simulink model "ViscoelasticBodies"  (R2025b)
settings: Solver=VariableStepAuto  StartTime=0.0  StopTime=10.0  RelTol=1e-3
undefined symbols (not defined in the file): sigbuilder_block
libraries: simulink x2
settings Model: Creator=ARDA  LastModifiedBy=carla
settings DebuggingCC: UnconnectedInputMsg=warning  UnconnectedOutputMsg=warning  UnconnectedLineMsg=warning
settings ModelReferenceCC: EnableRefExpFcnMdlSchedulingChecks=on
settings RTWCC: GPUComputeCapability=3.5  DLArmComputeVersion=19.05

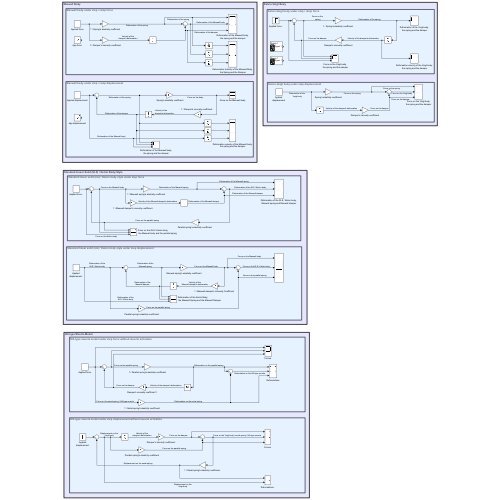
[thumbnail: Simulink's stored preview of the top-level diagram]
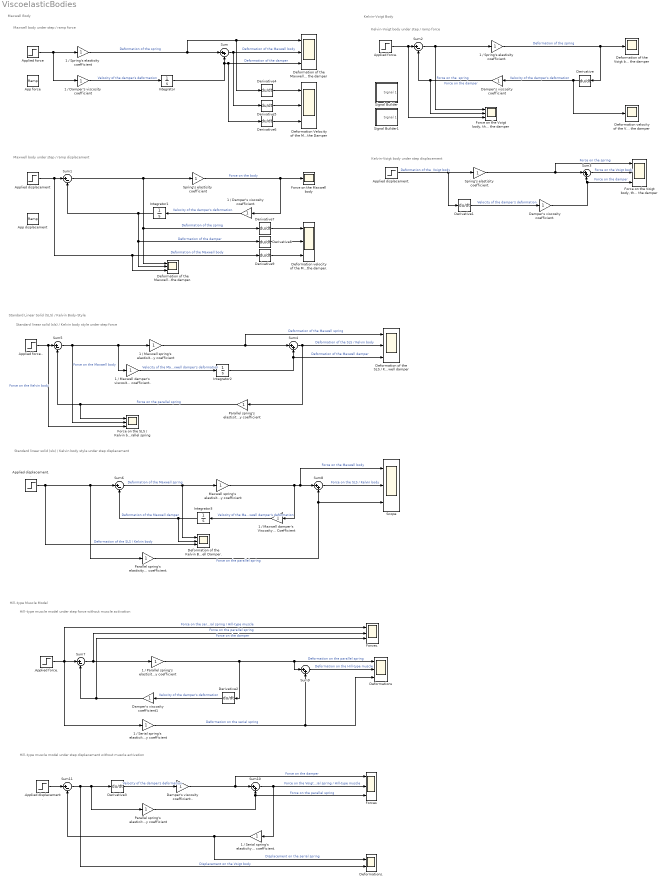
== system ViscoelasticBodies ==
  note: Hill-type Muscle Model
  note: Hill-type muscle model under step displacement without muscle activation
  note: Hill-type muscle model under step force without muscle activation
  note: Standard Linear Solid (SLS) / Kelvin Body-Style
  note: Standard linear solid (sls) / Kelvin body style under step displacement
  note: Standard linear solid (sls) / Kelvin body style under step force
  note: Kelvin-Voigt Body
  note: Kelvin-Voigt body under step displacement
  note: Kelvin-Voigt body under step / ramp force
  note: Maxwell Body
  note: Maxwell body under step / ramp displacement
  note: Maxwell body under step / ramp force
  .Applied displacement. : Step  SampleTime=0
  .Applied force. : Step  SampleTime=0
  1 / Damper's viscosity coefficient : Gain
  1 / Damper's viscosity coefficient. : Gain
  1 / Maxwell damper's Viscosity Coefficient : Gain
  1 / Maxwell damper's viscosity coefficient.. : Gain
  1 / Maxwell spring's elastisity coefficient : Gain
  1 / Parallel spring's elastisity coefficient : Gain
  1 / Serial spring's elasticity coefficient : Gain
  1 / Serial spring's elasticity coefficient. : Gain
  1 / Spring's elastisity coefficient : Gain
  1 / Spring's elastisity coefficient. : Gain
  App displacement : simulink/Sources/Ramp  slope=1  start=0  InitialOutput=0
  App force : simulink/Sources/Ramp  slope=1  start=0  InitialOutput=0
  Applied displacement. : Step  SampleTime=0
  Applied displacement.. : Step  SampleTime=0
  Applied displacement : Step  SampleTime=0
  Applied force : Step  SampleTime=0
  Applied force. : Step  SampleTime=0
  Applied force.. : Step  SampleTime=0
  Damper's viscosity coefficient : Gain
  Damper's viscosity coefficient. : Gain
  Damper's viscosity coefficient.. : Gain
  Damper's viscosity coefficient1 : Gain
  "Deformation Velocity of the Maxwell Body, the Spring and the Damper" : Scope  NumInputPorts=3
      settings: ActiveDisplayYMinimum=-1.7592186044415996E+13  ActiveDisplayYMaximum=1.58329674399744E+14
  "Deformation of the Kelvin Body, the Maxwell Spring and the Maxwell Damper." : Scope  NumInputPorts=3
      settings: ActiveDisplayYMinimum=-0.12499999999999997  ActiveDisplayYMaximum=1.125  DataLoggingVariableName=ScopeData8
  "Deformation of the Maxwell body, the spring and the damper" : Scope  NumInputPorts=3
      settings: ActiveDisplayYMinimum=-1.25  ActiveDisplayYMaximum=11.250000000000002
  "Deformation of the Maxwell body, the spring and the damper." : Scope  NumInputPorts=3
      settings: ActiveDisplayYMinimum=-0.12499999999999997  ActiveDisplayYMaximum=1.125  DataLoggingVariableName=ScopeData3
  "Deformation of the SLS / Kelvin body, Maxwell spring and Maxwell damper" : Scope  NumInputPorts=3
      settings: ActiveDisplayYMinimum=-0.12430568770609152  ActiveDisplayYMaximum=1.1187511893548239  DataLoggingVariableName=ScopeData6
  "Deformation of the Voigt body, the spring and the damper" : Scope
      settings: ActiveDisplayYMinimum=-0.12496582142586175  ActiveDisplayYMaximum=1.1246923928327561  DataLoggingVariableName=ScopeData2
  "Deformation velocity of the Maxwell body, the spring and the damper." : Scope  NumInputPorts=3
      settings: ActiveDisplayYMinimum=-1.7592186044417121E+13  ActiveDisplayYMaximum=1.5832967439974412E+14  DataLoggingVariableName=ScopeData2
  "Deformation velocity of the Voigt body, the spring and the damper" : Scope
      settings: ActiveDisplayYMinimum=-0.57803031764403257  ActiveDisplayYMaximum=0.67102285879629342
  Deformations : Scope  NumInputPorts=3
      settings: ActiveDisplayYMinimum=-0.24996582142586171  ActiveDisplayYMaximum=2.2496923928327561  DataLoggingVariableName=ScopeData2
  Deformations. : Scope  NumInputPorts=2
      settings: ActiveDisplayYMinimum=-0.12499999999999908  ActiveDisplayYMaximum=1.124999999999992
  Derivative{,1..9} (10 alike) : Derivative
  Force on the Maxwell body : Scope
      settings: ActiveDisplayYMinimum=-0.12499999999999997  ActiveDisplayYMaximum=1.125
  "Force on the SLS / Kelvin body, the Maxwell body and the parallel spring" : Scope  NumInputPorts=3
      settings: ActiveDisplayYMinimum=-0.125  ActiveDisplayYMaximum=1.125  DataLoggingVariableName=ScopeData7
  "Force on the Voigt body, the spring and the damper" : Scope  NumInputPorts=3
      settings: ActiveDisplayYMinimum=-0.66553  ActiveDisplayYMaximum=1.18506  DataLoggingVariableName=ScopeData4
  "Force on the Voigt body, the spring and the damper" : Scope  NumInputPorts=3
      settings: ActiveDisplayYMinimum=-1.7592186044416121E+13  ActiveDisplayYMaximum=1.5832967439974512E+14  DataLoggingVariableName=ScopeData5
  Forces : Scope  NumInputPorts=3
      settings: ActiveDisplayYMinimum=-0.12499999999999908  ActiveDisplayYMaximum=1.124999999999992  DataLoggingVariableName=ScopeData2
  Forces. : Scope  NumInputPorts=3
      settings: ActiveDisplayYMinimum=-0.12499999999999997  ActiveDisplayYMaximum=1.125  DataLoggingVariableName=ScopeData3
  Integrator{,1..3} (4 alike) : Integrator
  Maxwell spring's elastisity coefficient : Gain
  Parallel spring's elasticity coefficient : Gain
  Parallel spring's elastisity coefficient : Gain
  Parallel spring's elastisity coefficient. : Gain
  Scope : Scope  NumInputPorts=3
      settings: ActiveDisplayYMinimum=-0.24999999999999994  ActiveDisplayYMaximum=2.25  DataLoggingVariableName=ScopeData9
  Signal Builder : Subsystem  Tag=STV Subsys  LoadFcn=sigbuilder_block('load');  StartFcn=sigbuilder_block('start');  StopFcn=sigbuilder_block('stop');  ClipboardFcn=sigbuilder_block('clipboard');  mask(Sigbuilder block){tuvar=[0:10]}
      mask help: Simulink:masks:SigbuilderBlock_MD
      mask init:
      | if ~strcmp(get_param(bdroot(gcbh),'SimulationStatus'),'stopped') tuvar = sigbuilder_block('maskInit'); end
      settings: CopyFcn=sigbuilder_block('copy');  DeleteFcn=sigbuilder_block('delete');  ModelCloseFcn=sigbuilder_block('modelClose');  PreSaveFcn=sigbuilder_block('preSave');  PauseFcn=sigbuilder_block('pause');  ContinueFcn=sigbuilder_block('continue');  NameChangeFcn=sigbuilder_block('namechange');  OpenFcn=sigbuilder_block('open',[316.5 171.75 805.5 485.25 ]);  CloseFcn=sigbuilder_block('close');
      mask Display: plot(0, 0, 100, 100,[2, 2, 32, 32, 2], [68, 8, 8, 68, 68],[32, 2], [38, 38], [32, 19, 2],[53, 60, 44], [32, 17, 17, 2],[16, 16, 31, 31]);txt = getActiveGroup(gcbh);text(2, 100, txt,'verticalAlignment', 'top');
  Signal Builder1 : Subsystem  Tag=STV Subsys  LoadFcn=sigbuilder_block('load');  StartFcn=sigbuilder_block('start');  StopFcn=sigbuilder_block('stop');  ClipboardFcn=sigbuilder_block('clipboard');  mask(Sigbuilder block){tuvar=[0:10]}
      mask help: Simulink:masks:SigbuilderBlock_MD
      mask init:
      | if ~strcmp(get_param(bdroot(gcbh),'SimulationStatus'),'stopped') tuvar = sigbuilder_block('maskInit'); end
      settings: CopyFcn=sigbuilder_block('copy');  DeleteFcn=sigbuilder_block('delete');  ModelCloseFcn=sigbuilder_block('modelClose');  PreSaveFcn=sigbuilder_block('preSave');  PauseFcn=sigbuilder_block('pause');  ContinueFcn=sigbuilder_block('continue');  NameChangeFcn=sigbuilder_block('namechange');  OpenFcn=sigbuilder_block('open',[2397 1214.25 805.5 485.25 ]);  CloseFcn=sigbuilder_block('close');
      mask Display: plot(0, 0, 100, 100,[2, 2, 32, 32, 2], [68, 8, 8, 68, 68],[32, 2], [38, 38], [32, 19, 2],[53, 60, 44], [32, 17, 17, 2],[16, 16, 31, 31]);txt = getActiveGroup(gcbh);text(2, 100, txt,'verticalAlignment', 'top');
  Spring's elastisity coefficient : Gain
  Spring's elastisity coefficient. : Gain
  Sum{,3..4,8..10} (6 alike) : Sum  Inputs=|++
  Sum{1..2,5..7,11} (6 alike) : Sum  Inputs=|+-
  wires:
  Applied force/1 -> 1 / Damper's viscosity coefficient/1, 1 / Spring's elastisity coefficient/1
  1 / Damper's viscosity coefficient/1 -> Integrator/1  "Velocity of the damper's deformation"
  1 / Spring's elastisity coefficient/1 -> Derivative4/1, "Deformation of the Maxwell body, the spring and the damper"/1, Sum/1  "Deformation of the spring"
  Integrator/1 -> Derivative6/1, "Deformation of the Maxwell body, the spring and the damper"/3, Sum/2  "Deformation of the damper"
  Applied displacement/1 -> "Deformation of the Maxwell body, the spring and the damper."/3, Derivative9/1, Sum1/1  "Deformation of the Maxwell body"
  Sum1/1 -> Spring's elastisity coefficient/1, Derivative7/1, "Deformation of the Maxwell body, the spring and the damper."/1  "Deformation of the spring"
  Spring's elastisity coefficient/1 -> Force on the Maxwell body/1, 1 / Damper's viscosity coefficient./1  "Force on the body"
  1 / Damper's viscosity coefficient./1 -> Integrator1/1  "Velocity of the damper's deformation."
  Integrator1/1 -> Derivative8/1, "Deformation of the Maxwell body, the spring and the damper."/2, Sum1/2  "Deformation of the damper"
  Sum/1 -> Derivative5/1, "Deformation of the Maxwell body, the spring and the damper"/2  "Deformation of the Maxwell body"
  Applied force./1 -> "Force on the Voigt body, the spring and the damper"/3, Sum2/1
  Sum2/1 -> "Force on the Voigt body, the spring and the damper"/1, 1 / Spring's elastisity coefficient./1  "Force on the  spring"
  Damper's viscosity coefficient/1 -> Sum2/2, "Force on the Voigt body, the spring and the damper"/2  "Force on the damper"
  1 / Spring's elastisity coefficient./1 -> Derivative/1, "Deformation of the Voigt body, the spring and the damper"/1  "Deformation of the spring"
  Derivative/1 -> Damper's viscosity coefficient/1, "Deformation velocity of the Voigt body, the spring and the damper"/1  "Velocity of the damper's deformation"
  Applied displacement./1 -> Spring's elastisity coefficient./1, Derivative1/1  "Deformation of the  Voigt body"
  Derivative1/1 -> Damper's viscosity coefficient./1  "Velocity of the damper's deformation"
  Spring's elastisity coefficient./1 -> "Force on the Voigt body, the spring and the damper"/1, Sum3/1  "Force on the spring"
  Damper's viscosity coefficient./1 -> "Force on the Voigt body, the spring and the damper"/3, Sum3/2  "Force on the damper"
  Sum3/1 -> "Force on the Voigt body, the spring and the damper"/2  "Force on the Voigt body"
  Sum4/1 -> "Deformation of the SLS / Kelvin body, Maxwell spring and Maxwell damper"/2, Parallel spring's elastisity coefficient/1  "Deformation of the SLS / Kelvin body"
  Integrator2/1 -> "Deformation of the SLS / Kelvin body, Maxwell spring and Maxwell damper"/3, Sum4/2  "Deformation of the Maxwell damper"
  1 / Maxwell spring's elastisity coefficient/1 -> Sum4/1, "Deformation of the SLS / Kelvin body, Maxwell spring and Maxwell damper"/1  "Deformation of the Maxwell spring"
  1 / Maxwell damper's viscosity coefficient../1 -> Integrator2/1  "Velocity of the Maxwell damper's deformation"
  Sum5/1 -> "Force on the SLS / Kelvin body, the Maxwell body and the parallel spring"/2, 1 / Maxwell spring's elastisity coefficient/1, 1 / Maxwell damper's viscosity coefficient../1  "Force on the Maxwell body"
  Applied force../1 -> "Force on the SLS / Kelvin body, the Maxwell body and the parallel spring"/3, Sum5/1  "Force on the Kelvin body"
  Parallel spring's elastisity coefficient/1 -> "Force on the SLS / Kelvin body, the Maxwell body and the parallel spring"/1, Sum5/2  "Force on the parallel spring"
  Integrator3/1 -> "Deformation of the Kelvin Body, the Maxwell Spring and the Maxwell Damper."/2, Sum6/2  "Deformation of the Maxwell damper"
  1 / Maxwell damper's Viscosity Coefficient/1 -> Integrator3/1  "Velocity of the Maxwell damper's deformation"
  Maxwell spring's elastisity coefficient/1 -> Sum8/1, Scope/1, 1 / Maxwell damper's Viscosity Coefficient/1  "Force on the Maxwell body"
  Sum6/1 -> Maxwell spring's elastisity coefficient/1, "Deformation of the Kelvin Body, the Maxwell Spring and the Maxwell Damper."/1  "Deformation of the Maxwell spring"
  Applied displacement../1 -> Sum6/1, Parallel spring's elastisity coefficient./1, "Deformation of the Kelvin Body, the Maxwell Spring and the Maxwell Damper."/3  "Deformation of the SLS / Kelvin body"
  Parallel spring's elastisity coefficient./1 -> Scope/3, Sum8/2  "Force on the parallel spring"
  Sum8/1 -> Scope/2  "Force on the SLS / Kelvin body"
  Sum9/1 -> Deformations/2  "Deformation on the Hill-type muscle"
  Derivative2/1 -> Damper's viscosity coefficient1/1  "Velocity of the damper's deformation"
  1 / Parallel spring's elastisity coefficient/1 -> Sum9/1, Deformations/1, Derivative2/1  "Deformation on the parallel spring"
  1 / Serial spring's elasticity coefficient/1 -> Sum9/2, Deformations/3  "Deformation on the serial spring"
  Sum7/1 -> Forces./2, 1 / Parallel spring's elastisity coefficient/1  "Force on the parallel spring"
  Damper's viscosity coefficient1/1 -> Forces./3, Sum7/2  "Force on the damper"
  .Applied force./1 -> Forces./1, 1 / Serial spring's elasticity coefficient/1, Sum7/1  "Force on the serial spring / Hill-type muscle"
  Damper's viscosity coefficient../1 -> Forces/1, Sum10/1  "Force on the damper"
  Parallel spring's elasticity coefficient/1 -> Forces/3, Sum10/2  "Force on the parallel spring"
  .Applied displacement./1 -> Sum11/1
  Sum11/1 -> Derivative3/1, Parallel spring's elasticity coefficient/1, Deformations./2  "Displacement on the Voigt body"
  Derivative3/1 -> Damper's viscosity coefficient../1  "Velocity of the damper's deformation"
  Sum10/1 -> Forces/2, 1 / Serial spring's elasticity coefficient./1  "Force on the Voigt body / serial spring / Hill-type muscle"
  1 / Serial spring's elasticity coefficient./1 -> Sum11/2, Deformations./1  "Displacement on the serial spring"
  Derivative4/1 -> "Deformation Velocity of the Maxwell Body, the Spring and the Damper"/1
  Derivative5/1 -> "Deformation Velocity of the Maxwell Body, the Spring and the Damper"/2
  Derivative6/1 -> "Deformation Velocity of the Maxwell Body, the Spring and the Damper"/3
  Derivative8/1 -> "Deformation velocity of the Maxwell body, the spring and the damper."/2
  Derivative7/1 -> "Deformation velocity of the Maxwell body, the spring and the damper."/1
  Derivative9/1 -> "Deformation velocity of the Maxwell body, the spring and the damper."/3

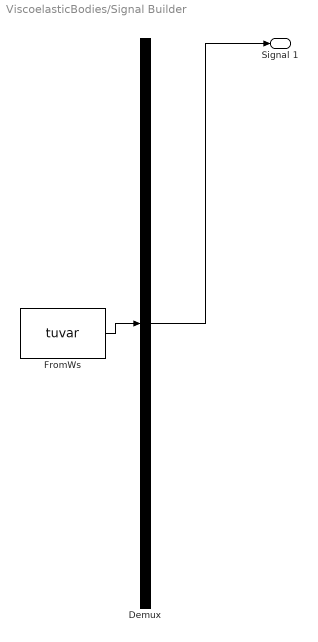
== system ViscoelasticBodies/Signal Builder ==
  Demux : Demux  Tag=STV Demux  Outputs=1
      settings: DisplayOption=none
  FromWs : FromWorkspace  Tag=STV FromWs  VariableName=tuvar
      SigBuilderData=|
      | common.afterFinalStr = 'Extrapolate'
      | common.sampleTime = 0
      | dataSet.timeRange = [0 10]
      | dataSet.name = 'Group 1'
      | sbobj.Groups.Name = 'Group 1'
      | sbobj.Groups.Signals.Name = 'Signal 1'
      | sbobj.Groups.Signals.XData = [0 1 1 2 2 10]
      | sbobj.Groups.Signals.YData = [0 0 1 1 0 0]
  Signal 1 : Outport  Tag=STV Outport
  wires:
  Demux/1 -> Signal 1/1
  FromWs/1 -> Demux/1

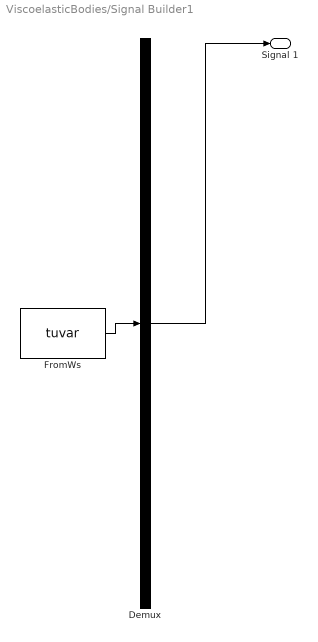
== system ViscoelasticBodies/Signal Builder1 ==
  Demux : Demux  Tag=STV Demux  Outputs=1
      settings: DisplayOption=none
  FromWs : FromWorkspace  Tag=STV FromWs  VariableName=tuvar
      SigBuilderData=|
      | common.afterFinalStr = 'Extrapolate'
      | common.sampleTime = 0
      | dataSet.timeRange = [0 10]
      | dataSet.name = 'Group 1'
      | sbobj.Groups.Name = 'Group 1'
      | sbobj.Groups.Signals.Name = 'Signal 1'
      | sbobj.Groups.Signals.XData = [0 1 1 2 2 10]
      | sbobj.Groups.Signals.YData = [0 0 0.265 1 0 0]
  Signal 1 : Outport  Tag=STV Outport
  wires:
  FromWs/1 -> Demux/1
  Demux/1 -> Signal 1/1
